simulink model "simA1"  (Simulink 8.3)
settings: Solver=ode45  StartTime=0.0  StopTime=10.0  RelTol=1e-3
settings Model: Creator=swami  LastModifiedBy=swami
settings DataIOCC: SignalLoggingSaveFormat=Dataset
settings DebuggingCC: UnderspecifiedInitializationDetection=Simplified  StateNameClashWarn=none
settings GRTTargetCC: CombineOutputUpdateFcns=on  GRTInterface=off

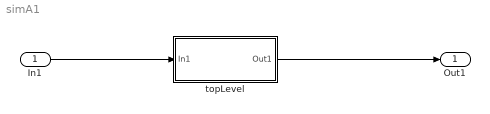
== system simA1 ==
  In1 : Inport
  topLevel : Subsystem
  Out1 : Outport
  wires:
  In1/1 -> topLevel/1(In1)
  topLevel/1(Out1) -> Out1/1

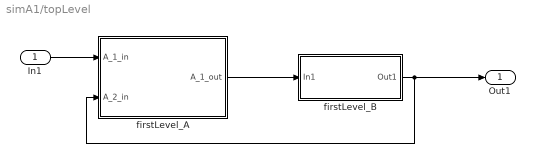
== system simA1/topLevel ==
  In1 : Inport
  firstLevel_A : Subsystem
  firstLevel_B : Subsystem
  Out1 : Outport
  wires:
  In1/1 -> firstLevel_A/1(A_1_in)
  firstLevel_A/1(A_1_out) -> firstLevel_B/1(In1)
  firstLevel_B/1(Out1) -> Out1/1, firstLevel_A/2(A_2_in)

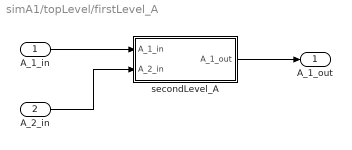
== system simA1/topLevel/firstLevel_A ==
  A_1_in : Inport
  A_2_in : Inport  Port=2
  secondLevel_A : Subsystem
  A_1_out : Outport
  wires:
  A_1_in/1 -> secondLevel_A/1(A_1_in)
  secondLevel_A/1(A_1_out) -> A_1_out/1
  A_2_in/1 -> secondLevel_A/2(A_2_in)

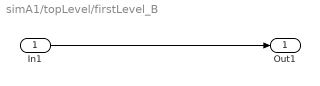
== system simA1/topLevel/firstLevel_B ==
  In1 : Inport
  Out1 : Outport
  wires:
  In1/1 -> Out1/1

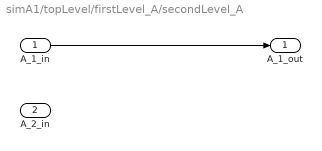
== system simA1/topLevel/firstLevel_A/secondLevel_A ==
  A_1_in : Inport
  A_2_in : Inport  Port=2
  A_1_out : Outport
  wires:
  A_1_in/1 -> A_1_out/1
